simulink subsystem "power_window_ECU"  (R2021a)
settings: Solver=VariableStepAuto  StartTime=0.0  StopTime=10.0  RelTol=1e-3
settings Model: Creator=achu  LastModifiedBy=achu

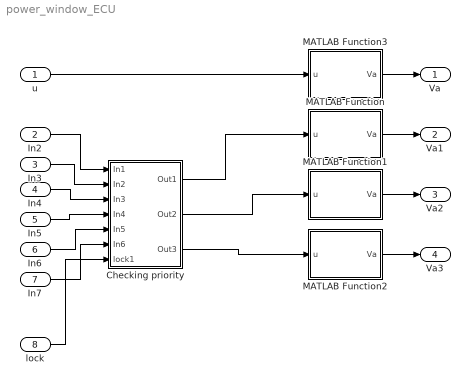
== system power_window_ECU ==
  u : Inport
  In2 : Inport  Port=2
  In3 : Inport  Port=3
  In4 : Inport  Port=4
  In5 : Inport  Port=5
  In6 : Inport  Port=6
  In7 : Inport  Port=7
  lock : Inport  Port=8
  Checking priority : Subsystem
  MATLAB Function : MATLAB Function  TreatAsAtomicUnit=on
  MATLAB Function1 : MATLAB Function  TreatAsAtomicUnit=on
  MATLAB Function2 : MATLAB Function  TreatAsAtomicUnit=on
  MATLAB Function3 : MATLAB Function  TreatAsAtomicUnit=on
  Va : Outport
  Va1 : Outport  Port=2
  Va2 : Outport  Port=3
  Va3 : Outport  Port=4
  wires:
  MATLAB Function/1(Va) -> Va1/1
  MATLAB Function2/1(Va) -> Va3/1
  In5/1 -> Checking priority/4(In4)
  u/1 -> MATLAB Function3/1(u)
  Checking priority/3(Out3) -> MATLAB Function2/1(u)
  In6/1 -> Checking priority/5(In5)
  Checking priority/1(Out1) -> MATLAB Function/1(u)
  In2/1 -> Checking priority/1(In1)
  MATLAB Function3/1(Va) -> Va/1
  In3/1 -> Checking priority/2(In2)
  MATLAB Function1/1(Va) -> Va2/1
  Checking priority/2(Out2) -> MATLAB Function1/1(u)
  In7/1 -> Checking priority/6(In6)
  In4/1 -> Checking priority/3(In3)
  lock/1 -> Checking priority/7(lock1)

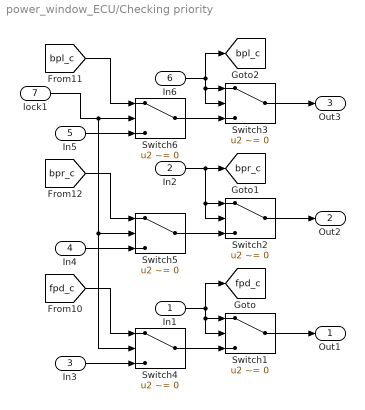
== system power_window_ECU/Checking priority ==
  In1 : Inport
  In2 : Inport  Port=2
  In3 : Inport  Port=3
  In4 : Inport  Port=4
  In5 : Inport  Port=5
  In6 : Inport  Port=6
  lock1 : Inport  Port=7
  Switch{1..6} (6 alike) : Switch  Criteria=u2 ~= 0
  Out1 : Outport
  Out2 : Outport  Port=2
  Out3 : Outport  Port=3
  tag scope: bpl_c=global, bpr_c=global, fpd_c=global
  wires:
  In2/1 -> Switch2/2, Switch2/1, [bpr_c]
  Switch2/1 -> Out2/1
  In3/1 -> Switch4/3
  Switch3/1 -> Out3/1
  In4/1 -> Switch5/3
  lock1/1 -> Switch6/2, Switch5/2, Switch4/2
  [fpd_c] -> Switch4/1
  Switch6/1 -> Switch3/3
  [bpl_c] -> Switch6/1
  In1/1 -> Switch1/2, Switch1/1, [fpd_c]
  Switch5/1 -> Switch2/3
  In5/1 -> Switch6/3
  [bpr_c] -> Switch5/1
  In6/1 -> Switch3/2, Switch3/1, [bpl_c]
  Switch1/1 -> Out1/1
  Switch4/1 -> Switch1/3

== matlab function power_window_ECU/MATLAB Function1 ==
  data: u input; Va output
function Va = fcn(u)
if (u==1)
    output=20;
elseif (u==-1)
    output=-20;
else
    output=0;
end
     
Va = output;

== matlab function power_window_ECU/MATLAB Function2 ==
  data: u input; Va output
function Va = fcn(u)
if (u==1)
    output=20;
elseif (u==-1)
    output=-20;
else
    output=0;
end
     
Va = output;

== matlab function power_window_ECU/MATLAB Function3 ==
  data: u input; Va output
function Va = fcn(u)
if (u==1)
    output=20;
elseif (u==-1)
    output=-20;
else
    output=0;
end
     
Va = output;

== matlab function power_window_ECU/MATLAB Function ==
  data: u input; Va output
function Va = fcn(u)
if (u==1)
    output=20;
elseif (u==-1)
    output=-20;
else
    output=0;
end
     
Va = output;
